simulink model "vehicle_progetto"  (R2022a)
settings: Solver=ode113  StartTime=0.0  StopTime=100.0  MinStep=1e-60  RelTol=1e-3
values from neighbouring files (symbols this model uses):
  a = 2    [vehicle_parameters.m]    (also in vehicle_parameters_v1.m = 1.3; vehicle_parameters_v1_sospensioni.m = 1.3)
  alpha = atan(w/(2*b))    [vehicle_parameters.m]    (also in vehicle_parameters_v1.m; vehicle_parameters_v1_sospensioni.m)
  b = 2.5    [vehicle_parameters.m]    (also in vehicle_parameters_v1.m = 1.8; vehicle_parameters_v1_sospensioni.m = 1.8)
  c = 0.13    [vehicle_parameters.m]
  ca = 0.5    [vehicle_parameters.m]    (also in vehicle_parameters_v1.m; vehicle_parameters_v1_sospensioni.m)
  cs = sqrt(2*ks*M)    [vehicle_parameters.m]    (also in vehicle_parameters_v1.m; vehicle_parameters_v1_sospensioni.m)
  h_gc = 0.15    [vehicle_parameters.m]    (also in vehicle_parameters_v1.m = 0.35; vehicle_parameters_v1_sospensioni.m = 0.35)
  Jx = 300    [vehicle_parameters.m]    (also in vehicle_parameters_v1.m; vehicle_parameters_v1_sospensioni.m)
  Jy = 500    [vehicle_parameters.m]    (also in vehicle_parameters_v1.m; vehicle_parameters_v1_sospensioni.m)
  Jz = 600    [vehicle_parameters.m]    (also in vehicle_parameters_v1.m; vehicle_parameters_v1_sospensioni.m)
  k_r = 1e4    (= 10000)    [vehicle_parameters.m]    (also in vehicle_parameters_v1.m = 2000000; vehicle_parameters_v1_sospensioni.m = 2000000)
  k_tu = 1500    [vehicle_parameters.m]    (also in vehicle_parameters_v1.m = 1500000; vehicle_parameters_v1_sospensioni.m = 1500000)
  k_tv = 400    [vehicle_parameters.m]    (also in vehicle_parameters_v1.m = 400000; vehicle_parameters_v1_sospensioni.m = 400000)
  ks = 40000    [vehicle_parameters.m]    (also in vehicle_parameters_v1.m = 39000; vehicle_parameters_v1_sospensioni.m = 9.75)
  L = sqrt(a^2+w^2 /4)    [vehicle_parameters.m]    (also in vehicle_parameters_v1.m; vehicle_parameters_v1_sospensioni.m)
  M = 1000    [vehicle_parameters.m]    (also in vehicle_parameters_v1.m = 1500; vehicle_parameters_v1_sospensioni.m = 1500)
  mu_dyn = 0.4    [vehicle_parameters.m]    (also in vehicle_parameters_v1.m = 0.2; vehicle_parameters_v1_sospensioni.m = 0.2)
  mu_st = 0.8    [vehicle_parameters.m]    (also in vehicle_parameters_v1.m; vehicle_parameters_v1_sospensioni.m)
  r = 0.2    [vehicle_parameters.m]    (also in vehicle_parameters_v1.m = 0.3; vehicle_parameters_v1_sospensioni.m = 0.3)
  R = sqrt(b^2+w^2 /4)    [vehicle_parameters.m]    (also in vehicle_parameters_v1.m; vehicle_parameters_v1_sospensioni.m)
  S = 0.13*0.2    (= 0.026)    [vehicle_parameters.m]
  theta = atan(w/(2*a))    [vehicle_parameters.m]    (also in vehicle_parameters_v1.m; vehicle_parameters_v1_sospensioni.m)
settings Model: Creator=jackrip  LastModifiedBy=jackrip

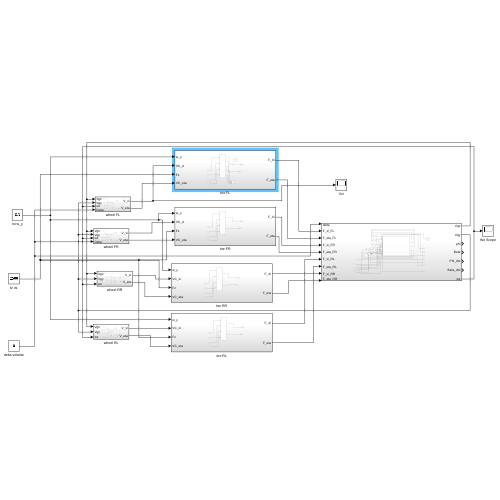
[thumbnail: Simulink's stored preview of the top-level diagram]
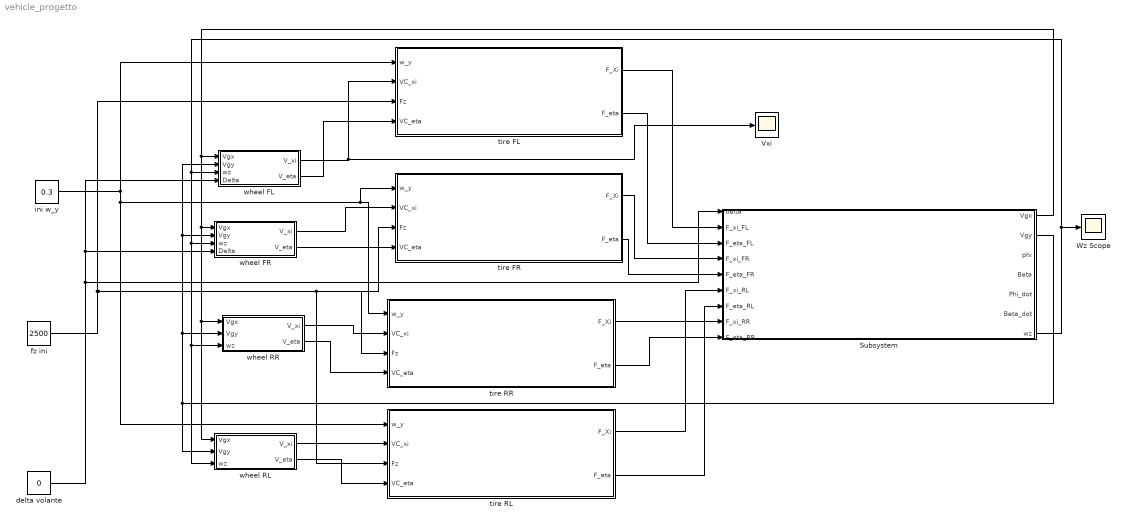
== system vehicle_progetto ==
  Subsystem : Subsystem
  Vxi : Scope
  Wz Scope : Scope
  delta volante : Constant  Value=0
  fz ini : Constant  Value=2500
  ini w_y : Constant  Value=0.3
  tire FL : Subsystem
  tire FR : Subsystem
  tire RL : Subsystem
  tire RR : Subsystem
  wheel FL : Subsystem
  wheel FR : Subsystem
  wheel RL : Subsystem
  wheel RR : Subsystem
  wires:
  wheel FL/1(V_xi) -> Vxi/1, tire FL/2(VC_xi)
  wheel FL/2(V_eta) -> tire FL/4(VC_eta)
  tire FL/1(F_Xi) -> Subsystem/2(F_xi_FL)
  tire FL/2(F_eta) -> Subsystem/3(F_eta_FL)
  tire RL/1(F_Xi) -> Subsystem/6(F_xi_RL)
  tire RL/2(F_eta) -> Subsystem/7(F_eta_RL)
  tire RR/1(F_Xi) -> Subsystem/8(F_xi_RR)
  tire RR/2(F_eta) -> Subsystem/9(F_eta_RR)
  tire FR/1(F_Xi) -> Subsystem/4(F_xi_FR)
  tire FR/2(F_eta) -> Subsystem/5(F_eta_FR)
  wheel FR/1(V_xi) -> tire FR/2(VC_xi)
  wheel FR/2(V_eta) -> tire FR/4(VC_eta)
  wheel RL/1(V_xi) -> tire RL/2(VC_xi)
  wheel RR/1(V_xi) -> tire RR/2(VC_xi)
  wheel RR/2(V_eta) -> tire RR/4(VC_eta)
  wheel RL/2(V_eta) -> tire RL/4(VC_eta)
  Subsystem/1(Vgx) -> wheel RL/1(Vgx), wheel RR/1(Vgx), wheel FR/1(Vgx), wheel FL/1(Vgx)
  Subsystem/2(Vgy) -> wheel FL/2(Vgy), wheel FR/2(Vgy), wheel RR/2(Vgy), wheel RL/2(Vgy)
  Subsystem/7(wz) -> Wz Scope/1, wheel RL/3(wz), wheel RR/3(wz), wheel FR/3(wz), wheel FL/3(wz)
  ini w_y/1 -> tire RL/1(w_y), tire RR/1(w_y), tire FR/1(w_y), tire FL/1(w_y)
  fz ini/1 -> tire RL/3(Fz), tire FR/3(Fz), tire RR/3(Fz), tire FL/3(Fz)
  delta volante/1 -> wheel FL/4(Delta), wheel FR/4(Delta), Subsystem/1(delta)

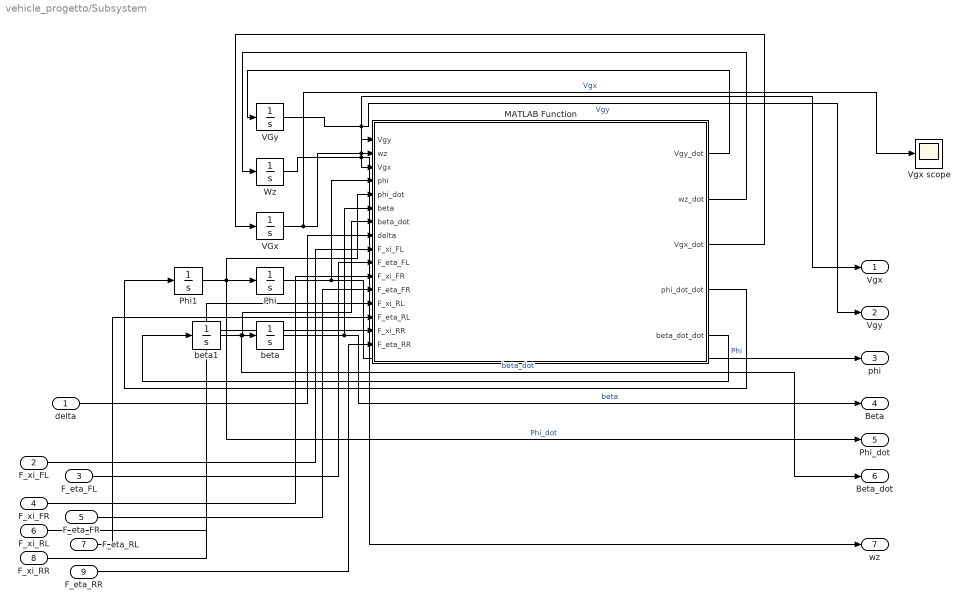
== system vehicle_progetto/Subsystem ==
  delta : Inport
  F_xi_FL : Inport  Port=2
  F_eta_FL : Inport  Port=3
  F_xi_FR : Inport  Port=4
  F_eta_FR : Inport  Port=5
  F_xi_RL : Inport  Port=6
  F_eta_RL : Inport  Port=7
  F_xi_RR : Inport  Port=8
  F_eta_RR : Inport  Port=9
  MATLAB Function : MATLAB Function  TreatAsAtomicUnit=on
  Phi : Integrator
  Phi1 : Integrator
  VGx : Integrator  InitialCondition=0.055
  VGy : Integrator
  Vgx scope : Scope
  Wz : Integrator
  beta : Integrator
  beta1 : Integrator
  Vgx : Outport
  Vgy : Outport  Port=2
  phi : Outport  Port=3
  Beta : Outport  Port=4
  Phi_dot : Outport  Port=5
  Beta_dot : Outport  Port=6
  wz : Outport  Port=7
  wires:
  Phi1/1 -> Phi_dot/1, MATLAB Function/5(phi_dot), Phi/1  "Phi_dot"
  MATLAB Function/1(Vgy_dot) -> VGy/1
  VGy/1 -> Vgy/1, MATLAB Function/1(Vgy)  "Vgy"
  MATLAB Function/2(wz_dot) -> Wz/1
  Wz/1 -> wz/1, MATLAB Function/2(wz)
  MATLAB Function/3(Vgx_dot) -> VGx/1
  VGx/1 -> Vgx scope/1, Vgx/1, MATLAB Function/3(Vgx)  "Vgx"
  MATLAB Function/4(phi_dot_dot) -> Phi1/1
  Phi/1 -> phi/1, MATLAB Function/4(phi)  "Phi"
  beta1/1 -> MATLAB Function/7(beta_dot), beta/1, Beta_dot/1  "beta_dot"
  MATLAB Function/5(beta_dot_dot) -> beta1/1
  beta/1 -> Beta/1, MATLAB Function/6(beta)  "beta"
  delta/1 -> MATLAB Function/8(delta)
  F_xi_FL/1 -> MATLAB Function/9(F_xi_FL)
  F_eta_FL/1 -> MATLAB Function/10(F_eta_FL)
  F_xi_FR/1 -> MATLAB Function/11(F_xi_FR)
  F_eta_FR/1 -> MATLAB Function/12(F_eta_FR)
  F_xi_RL/1 -> MATLAB Function/13(F_xi_RL)
  F_eta_RL/1 -> MATLAB Function/14(F_eta_RL)
  F_xi_RR/1 -> MATLAB Function/15(F_xi_RR)
  F_eta_RR/1 -> MATLAB Function/16(F_eta_RR)

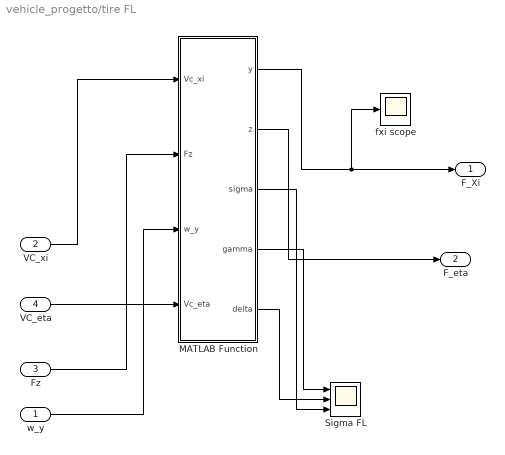
== system vehicle_progetto/tire FL ==
  w_y : Inport
  VC_xi : Inport  Port=2
  Fz : Inport  Port=3
  VC_eta : Inport  Port=4
  MATLAB Function : MATLAB Function  TreatAsAtomicUnit=on
  Sigma FL : Scope  NumInputPorts=3
  fxi scope : Scope
  F_Xi : Outport
  F_eta : Outport  Port=2
  wires:
  MATLAB Function/1(y) -> fxi scope/1, F_Xi/1
  VC_xi/1 -> MATLAB Function/1(Vc_xi)
  Fz/1 -> MATLAB Function/2(Fz)
  w_y/1 -> MATLAB Function/3(w_y)
  MATLAB Function/2(z) -> F_eta/1
  VC_eta/1 -> MATLAB Function/4(Vc_eta)
  MATLAB Function/3(sigma) -> Sigma FL/3
  MATLAB Function/4(gamma) -> Sigma FL/1
  MATLAB Function/5(delta) -> Sigma FL/2

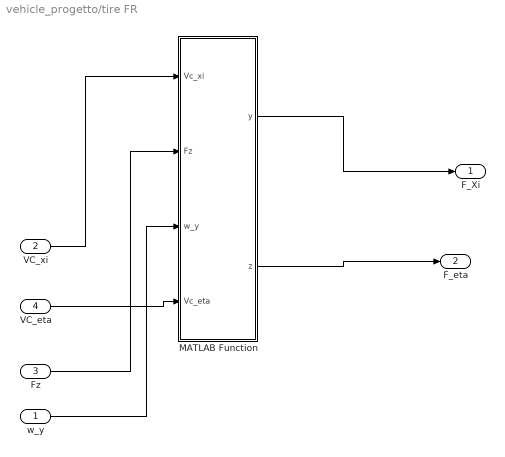
== system vehicle_progetto/tire FR ==
  w_y : Inport
  VC_xi : Inport  Port=2
  Fz : Inport  Port=3
  VC_eta : Inport  Port=4
  MATLAB Function : MATLAB Function  TreatAsAtomicUnit=on
  F_Xi : Outport
  F_eta : Outport  Port=2
  wires:
  MATLAB Function/1(y) -> F_Xi/1
  VC_xi/1 -> MATLAB Function/1(Vc_xi)
  Fz/1 -> MATLAB Function/2(Fz)
  w_y/1 -> MATLAB Function/3(w_y)
  MATLAB Function/2(z) -> F_eta/1
  VC_eta/1 -> MATLAB Function/4(Vc_eta)

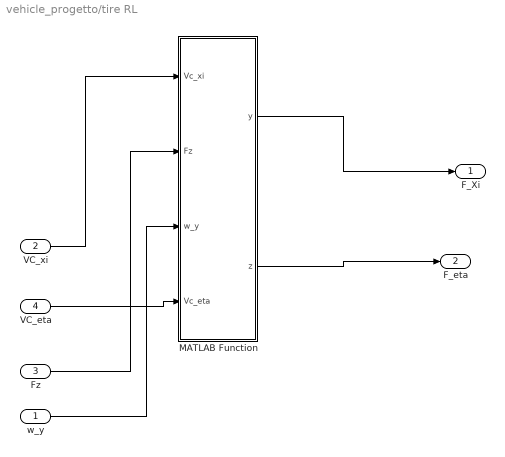
== system vehicle_progetto/tire RL ==
  w_y : Inport
  VC_xi : Inport  Port=2
      settings: AttributesFormatString=|
      | Velocità Del centro della ruota diretta lungo l'asse della ruota
      | Se la macchina stesse andando dritta sarebbe uguale a vgx
  Fz : Inport  Port=3
  VC_eta : Inport  Port=4
  MATLAB Function : MATLAB Function  TreatAsAtomicUnit=on
  F_Xi : Outport
  F_eta : Outport  Port=2
  wires:
  MATLAB Function/1(y) -> F_Xi/1
  VC_xi/1 -> MATLAB Function/1(Vc_xi)
  Fz/1 -> MATLAB Function/2(Fz)
  w_y/1 -> MATLAB Function/3(w_y)
  MATLAB Function/2(z) -> F_eta/1
  VC_eta/1 -> MATLAB Function/4(Vc_eta)

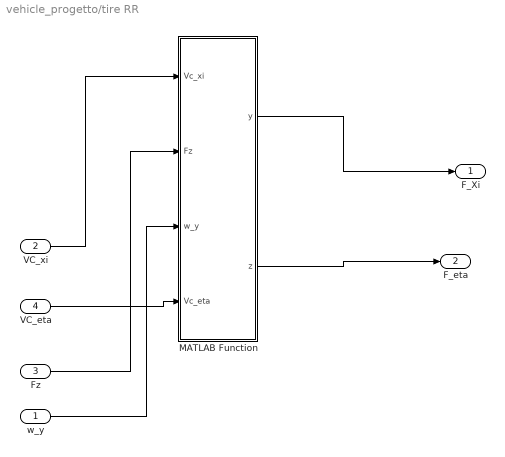
== system vehicle_progetto/tire RR ==
  w_y : Inport
  VC_xi : Inport  Port=2
  Fz : Inport  Port=3
  VC_eta : Inport  Port=4
  MATLAB Function : MATLAB Function  TreatAsAtomicUnit=on
  F_Xi : Outport
  F_eta : Outport  Port=2
  wires:
  MATLAB Function/1(y) -> F_Xi/1
  VC_xi/1 -> MATLAB Function/1(Vc_xi)
  Fz/1 -> MATLAB Function/2(Fz)
  w_y/1 -> MATLAB Function/3(w_y)
  MATLAB Function/2(z) -> F_eta/1
  VC_eta/1 -> MATLAB Function/4(Vc_eta)

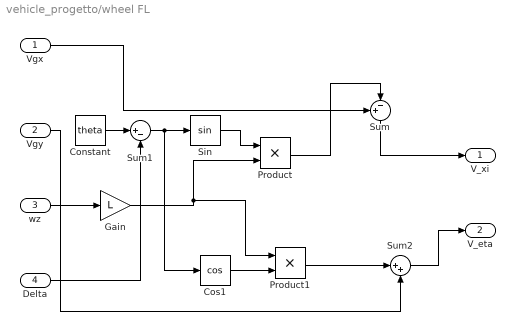
== system vehicle_progetto/wheel FL ==
  Vgx : Inport
  Vgy : Inport  Port=2
  wz : Inport  Port=3
  Delta : Inport  Port=4
  Constant : Constant  Value=theta
  Cos1 : Trigonometry  Operator=cos
  Gain : Gain  Gain=L
  Product : Product
  Product1 : Product
  Sin : Trigonometry
  Sum : Sum  Inputs=+-|
  Sum1 : Sum  Inputs=|+-
  Sum2 : Sum  Inputs=|++
  V_xi : Outport
  V_eta : Outport  Port=2
  wires:
  Vgx/1 -> Sum/1
  wz/1 -> Gain/1
  Sin/1 -> Product/1
  Constant/1 -> Sum1/1
  Sum1/1 -> Cos1/1, Sin/1
  Delta/1 -> Sum1/2
  Product/1 -> Sum/2
  Sum/1 -> V_xi/1
  Cos1/1 -> Product1/2
  Gain/1 -> Product/2, Product1/1
  Product1/1 -> Sum2/1
  Sum2/1 -> V_eta/1
  Vgy/1 -> Sum2/2

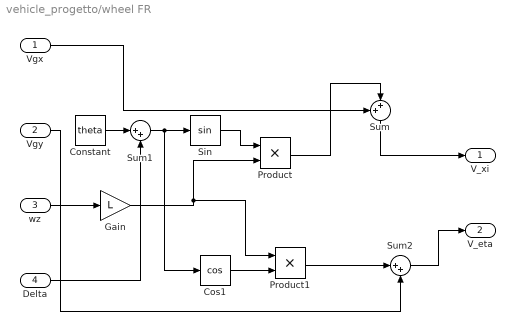
== system vehicle_progetto/wheel FR ==
  Vgx : Inport
  Vgy : Inport  Port=2
  wz : Inport  Port=3
  Delta : Inport  Port=4
  Constant : Constant  Value=theta
  Cos1 : Trigonometry  Operator=cos
  Gain : Gain  Gain=L
  Product : Product
  Product1 : Product
  Sin : Trigonometry
  Sum : Sum  Inputs=++|
  Sum1 : Sum  Inputs=|++
  Sum2 : Sum  Inputs=|++
  V_xi : Outport
  V_eta : Outport  Port=2
  wires:
  Vgx/1 -> Sum/1
  wz/1 -> Gain/1
  Sin/1 -> Product/1
  Constant/1 -> Sum1/1
  Sum1/1 -> Cos1/1, Sin/1
  Delta/1 -> Sum1/2
  Product/1 -> Sum/2
  Sum/1 -> V_xi/1
  Cos1/1 -> Product1/2
  Gain/1 -> Product/2, Product1/1
  Product1/1 -> Sum2/1
  Sum2/1 -> V_eta/1
  Vgy/1 -> Sum2/2

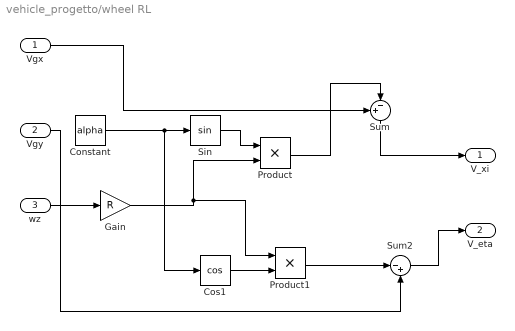
== system vehicle_progetto/wheel RL ==
  Vgx : Inport
  Vgy : Inport  Port=2
  wz : Inport  Port=3
  Constant : Constant  Value=alpha
  Cos1 : Trigonometry  Operator=cos
  Gain : Gain  Gain=R
  Product : Product
  Product1 : Product
  Sin : Trigonometry
  Sum : Sum  Inputs=+-|
  Sum2 : Sum  Inputs=|-+
  V_xi : Outport
  V_eta : Outport  Port=2
  wires:
  Vgx/1 -> Sum/1
  wz/1 -> Gain/1
  Sin/1 -> Product/1
  Constant/1 -> Cos1/1, Sin/1
  Product/1 -> Sum/2
  Sum/1 -> V_xi/1
  Cos1/1 -> Product1/2
  Gain/1 -> Product/2, Product1/1
  Product1/1 -> Sum2/1
  Sum2/1 -> V_eta/1
  Vgy/1 -> Sum2/2

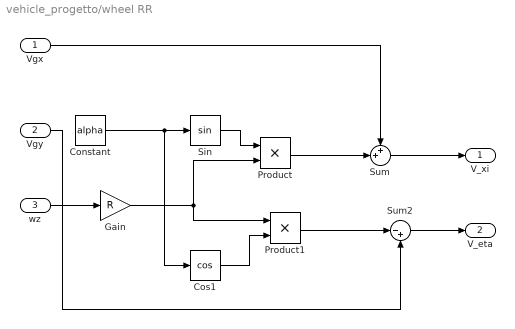
== system vehicle_progetto/wheel RR ==
  Vgx : Inport
  Vgy : Inport  Port=2
  wz : Inport  Port=3
  Constant : Constant  Value=alpha
  Cos1 : Trigonometry  Operator=cos
  Gain : Gain  Gain=R
  Product : Product
  Product1 : Product
  Sin : Trigonometry
  Sum : Sum  Inputs=++|
  Sum2 : Sum  Inputs=|-+
  V_xi : Outport
  V_eta : Outport  Port=2
  wires:
  Vgx/1 -> Sum/1
  wz/1 -> Gain/1
  Sin/1 -> Product/1
  Constant/1 -> Cos1/1, Sin/1
  Product/1 -> Sum/2
  Sum/1 -> V_xi/1
  Cos1/1 -> Product1/2
  Gain/1 -> Product/2, Product1/1
  Product1/1 -> Sum2/1
  Sum2/1 -> V_eta/1
  Vgy/1 -> Sum2/2

== matlab function vehicle_progetto/tire RR/MATLAB Function ==
  data: Vc_xi input; y output; Fz input; w_y input; r parameter; c parameter; mu_st parameter; k_r parameter; mu_dyn parameter; S parameter; k_tv parameter; k_tu parameter; z output; Vc_eta input
function [y,z] = fcn(Vc_xi, Fz, w_y,r, c, mu_st, k_r, mu_dyn, S, k_tv, k_tu, Vc_eta)
sigma=(Vc_xi-w_y*r)/Vc_xi;
gamma = Vc_eta/Vc_xi;
delta = r*2*sqrt(k_tu^2*sigma^2+k_tv^2*gamma^2)/(c*mu_st*k_r);
if delta>1
    delta=1;
end
F_xi = -sign(Vc_xi-w_y*r)*mu_st*Fz*(6*abs(sigma)/(sqrt(sigma^2+gamma^2))*mu_dyn/mu_st*(0.5-1/3*delta)*(delta)^2+S*k_tu*c/(2*mu_st*Fz)*(delta-1)^2*abs(sigma));
F_eta = mu_st*Fz*(6*gamma/(sqrt(sigma^2+gamma^2))*mu_dyn/mu_st*(0.5-1/3*delta)*(delta)^2+S*k_tv*c/(2*mu_st*Fz)*(delta-1)^2*gamma);
y = F_xi;
z = F_eta;

== matlab function vehicle_progetto/tire FR/MATLAB Function ==
  data: Vc_xi input; y output; Fz input; w_y input; r parameter; c parameter; mu_st parameter; k_r parameter; mu_dyn parameter; S parameter; k_tv parameter; k_tu parameter; z output; Vc_eta input
function [y,z] = fcn(Vc_xi, Fz, w_y,r, c, mu_st, k_r, mu_dyn, S, k_tv, k_tu, Vc_eta)
sigma=(Vc_xi-w_y*r)/Vc_xi;
gamma = Vc_eta/Vc_xi;
delta = r*2*sqrt(k_tu^2*sigma^2+k_tv^2*gamma^2)/(c*mu_st*k_r);
if delta>1
    delta=1;
end
F_xi = -sign(Vc_xi-w_y*r)*mu_st*Fz*(6*abs(sigma)/(sqrt(sigma^2+gamma^2))*mu_dyn/mu_st*(0.5-1/3*delta)*(delta)^2+S*k_tu*c/(2*mu_st*Fz)*(delta-1)^2*abs(sigma));
F_eta = mu_st*Fz*(6*gamma/(sqrt(sigma^2+gamma^2))*mu_dyn/mu_st*(0.5-1/3*delta)*(delta)^2+S*k_tv*c/(2*mu_st*Fz)*(delta-1)^2*gamma);
y = F_xi;
z = F_eta;

== matlab function vehicle_progetto/tire RL/MATLAB Function ==
  data: Vc_xi input; y output; Fz input; w_y input; r parameter; c parameter; mu_st parameter; k_r parameter; mu_dyn parameter; S parameter; k_tv parameter; k_tu parameter; z output; Vc_eta input
function [y,z] = fcn(Vc_xi, Fz, w_y,r, c, mu_st, k_r, mu_dyn, S, k_tv, k_tu, Vc_eta)
sigma=(Vc_xi-w_y*r)/Vc_xi;
gamma = Vc_eta/Vc_xi;
delta = r*2*sqrt(k_tu^2*sigma^2+k_tv^2*gamma^2)/(c*mu_st*k_r);
if delta>1
    delta=1;
end
F_xi = -sign(Vc_xi-w_y*r)*mu_st*Fz*(6*abs(sigma)/(sqrt(sigma^2+gamma^2))*mu_dyn/mu_st*(0.5-1/3*delta)*(delta)^2+S*k_tu*c/(2*mu_st*Fz)*(delta-1)^2*abs(sigma));
F_eta = mu_st*Fz*(6*gamma/(sqrt(sigma^2+gamma^2))*mu_dyn/mu_st*(0.5-1/3*delta)*(delta)^2+S*k_tv*c/(2*mu_st*Fz)*(delta-1)^2*gamma);
y = F_xi;
z = F_eta;

== matlab function vehicle_progetto/tire FL/MATLAB Function ==
  data: Vc_xi input; y output; Fz input; w_y input; r parameter; c parameter; mu_st parameter; k_r parameter; mu_dyn parameter; S parameter; k_tv parameter; k_tu parameter; z output; Vc_eta input; sigma output; gamma output; delta output
function [y,z,sigma,gamma,delta] = fcn(Vc_xi, Fz, w_y,r, c, mu_st, k_r, mu_dyn, S, k_tv, k_tu, Vc_eta)
sigma=(Vc_xi-w_y*r)/Vc_xi;
gamma = Vc_eta/Vc_xi;
delta = r*2*sqrt(k_tu^2*sigma^2+k_tv^2*gamma^2)/(c*mu_st*k_r);
if delta>1
    delta=1;
end
F_xi = -sign(Vc_xi-w_y*r)*mu_st*Fz*(6*abs(sigma)/(sqrt(sigma^2+gamma^2))*mu_dyn/mu_st*(0.5-1/3*delta)*(delta)^2+S*k_tu*c/(2*mu_st*Fz)*(delta-1)^2*abs(sigma));
F_eta = mu_st*Fz*(6*gamma/(sqrt(sigma^2+gamma^2))*mu_dyn/mu_st*(0.5-1/3*delta)*(delta)^2+S*k_tv*c/(2*mu_st*Fz)*(delta-1)^2*gamma);
y = F_xi;
z = F_eta;

== matlab function vehicle_progetto/Subsystem/MATLAB Function ==
  data: Vgy input; Vgy_dot output; wz input; Vgx input; phi input; phi_dot input; beta input; beta_dot input; delta input; F_xi_FL input; F_eta_FL input; F_xi_FR input; F_eta_FR input; F_xi_RL input; F_eta_RL input; F_xi_RR input; F_eta_RR input; wz_dot output; Vgx_dot output; phi_dot_dot output; beta_dot_dot output; M parameter; a parameter; b parameter; h_gc parameter; Jx parameter; Jy parameter; Jz parameter; ks parameter; cs parameter; ca parameter
function [Vgy_dot, wz_dot, Vgx_dot, phi_dot_dot, beta_dot_dot] = fcn(Vgy, wz, Vgx, phi, phi_dot, beta, beta_dot, delta, F_xi_FL, F_eta_FL,  F_xi_FR, F_eta_FR,  F_xi_RL, F_eta_RL, F_xi_RR, F_eta_RR, M, a, b, h_gc, Jx, Jy, Jz, ks, cs,ca)

F_air=0;%ca*Vgx^2;
Fy = (F_eta_RL + F_eta_RR)+ (F_eta_FL + F_eta_FR)*cos(delta) + (F_xi_FL + F_xi_FR)*sin(delta); %data dalla trazione delle ruote

% disp(F_eta_RL)
% disp(F_eta_RR)
% disp(F_eta_FR)
% disp(F_xi_FL)
% disp(F_xi_FR)
% disp(Fy)
% disp(M)
% disp(wz)
% disp(Vgx)

Vgy_dot = Fy/M - wz*Vgx ;
% disp(Vgy_dot)

Mgz = -(F_eta_RL + F_eta_RR)*b+(F_eta_FL + F_eta_FR)*cos(delta)*a*(F_eta_FL + F_eta_FR)*sin(delta)*a;
wz_dot = Mgz/Jz;
Fx = (F_xi_RL + F_xi_RR)+(F_xi_FL + F_xi_FR)*cos(delta)-(F_eta_FL + F_eta_FR)*sin(delta);
Vgx_dot = Fx/M -F_air/M*sign(Vgx);
phi_dot_dot = -ks*phi/Jx -cs*phi_dot/Jx + Fy*h_gc/Jx;
My = Fx*h_gc;
beta_dot_dot = -ks*beta/Jy -cs*beta_dot/Jy + My/Jy;
